simulink model "MRAC3sim"  (R2019a)
settings: Solver=VariableStepAuto  StartTime=0.0  StopTime=20  RelTol=1e-3
values from neighbouring files (symbols this model uses):
  a0 = 3    [Gradient_instant_cost.m]    (also in Gradient_integral_cost.m; MRAC.m = 3+n(1); MRAC2.m = 1+n(1); MRAC3.m = 1)
  a1 = 2    [Gradient_instant_cost.m]    (also in Gradient_integral_cost.m; MRAC.m = 5+n(2); MRAC2.m = 5+n(2); MRAC3.m = 3)
  b0 = 1    [Gradient_instant_cost.m]    (also in Gradient_integral_cost.m; MRAC.m = 7+n(3); MRAC2.m = 3+n(3); MRAC3.m = 3)
  gamma = diag([0.01,0.01,0.005,0.005])    [MRAC3.m]    (also in Parameter_estimation.m = 10*i; Untitled2.m = 10; Untitled34.m = 1; Untitled9.m = 1)
  Km = 1    [Untitled2.m]
  Kp = 1    [MRAC3.m]    (also in Untitled2.m)
  lambda = [lambda1; lambda0]    [Gradient_instant_cost.m]    (also in Gradient_integral_cost.m; PureLSQ.m; Untitled2.m = 10; Untitled34.m = 1)
  w0 = 3    [MRAC.m]    (also in MRAC2.m; Untitled2.m = 1; Untitled5.m = 2; Untitled9.m = 1)
settings Model: Creator=Student  LastModifiedBy=Student

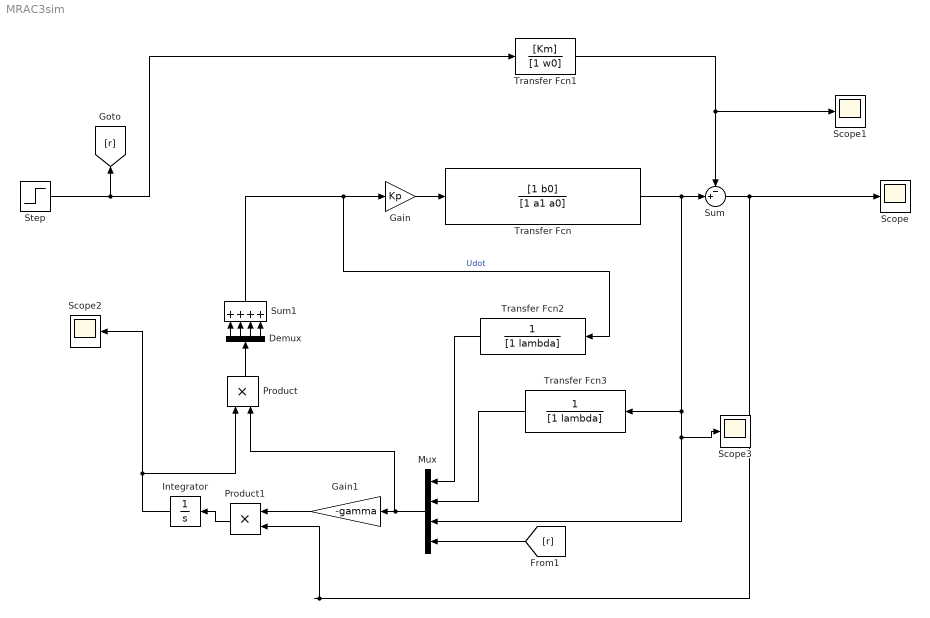
== system MRAC3sim ==
  Demux : Demux
  Gain : Gain  Gain=Kp
  Gain1 : Gain  Gain=-gamma
  Integrator : Integrator
  Mux : Mux
  Product : Product
  Product1 : Product
  Scope{,1..3} (4 alike) : Scope
  Step : Step  Time=0  SampleTime=0
  Sum : Sum  Inputs=-+|
  Sum1 : Sum  Inputs=4
  Transfer Fcn : TransferFcn  Numerator=[1 b0]  Denominator=[1 a1 a0]
  Transfer Fcn1 : TransferFcn  Numerator=[Km]  Denominator=[1 w0]
  Transfer Fcn2 : TransferFcn  Denominator=[1 lambda]
  Transfer Fcn3 : TransferFcn  Denominator=[1 lambda]
  wires:
  Transfer Fcn2/1 -> Mux/1
  Mux/1 -> Product/2, Gain1/1
  Transfer Fcn3/1 -> Mux/2
  Integrator/1 -> Scope2/1, Product/1
  Product/1 -> Demux/1
  Demux/1 -> Sum1/1
  Demux/2 -> Sum1/2
  Demux/3 -> Sum1/3
  Demux/4 -> Sum1/4
  Step/1 -> [r], Transfer Fcn1/1
  Sum/1 -> Scope/1, Product1/2
  Gain1/1 -> Product1/1
  Product1/1 -> Integrator/1
  Transfer Fcn1/1 -> Sum/1, Scope1/1
  [r] -> Mux/4
  Sum1/1 -> Transfer Fcn2/1, Gain/1  "Udot"
  Gain/1 -> Transfer Fcn/1
  Transfer Fcn/1 -> Scope3/1, Mux/3, Transfer Fcn3/1, Sum/2
